simulink library "sensor_processing_libs"  (R2016b)
settings: Solver=VariableStepAuto  StartTime=0.0  StopTime=10.0  RelTol=1e-3
undefined symbols (not defined in the file or in its folder): fsw_params
settings Model: Creator=taylorreynolds  LastModifiedBy=Taylor

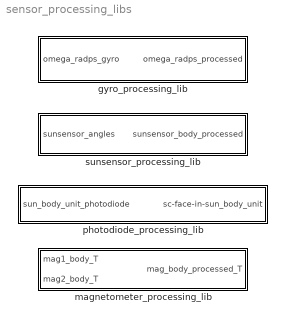
== system sensor_processing_libs ==
  gyro_processing_lib : Subsystem
  magnetometer_processing_lib : Subsystem
  photodiode_processing_lib : Subsystem
  sunsensor_processing_lib : Subsystem

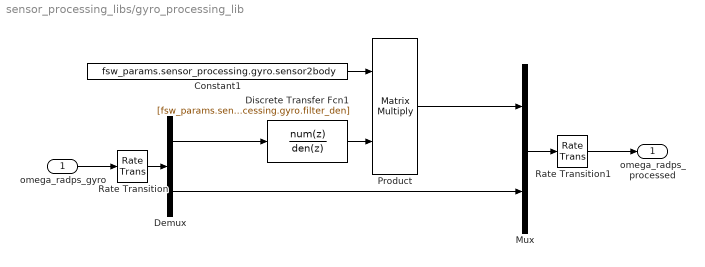
== system sensor_processing_libs/gyro_processing_lib ==
  omega_radps_gyro : Inport
  Constant1 : Constant  Value=fsw_params.sensor_processing.gyro.sensor2body  OutDataTypeStr=single  SampleTime=fsw_params.sensor_processing.gyro.sample_time_s
  Demux : Demux  Outputs=[3 1]
  Discrete Transfer Fcn1 : DiscreteTransferFcn  Numerator=[fsw_params.sensor_processing.gyro.filter_num]  Denominator=[1 fsw_params.sensor_processing.gyro.filter_den]
  Mux : Mux  Inputs=[3 1]
  Product : Product  Multiplication=Matrix(*)
  Rate Transition : RateTransition  OutPortSampleTime=fsw_params.sensor_processing.gyro.sample_time_s
  Rate Transition1 : RateTransition
  omega_radps_processed : Outport
  wires:
  omega_radps_gyro/1 -> Rate Transition/1
  Demux/1 -> Discrete Transfer Fcn1/1
  Constant1/1 -> Product/1
  Demux/2 -> Mux/2
  Discrete Transfer Fcn1/1 -> Product/2
  Rate Transition/1 -> Demux/1
  Rate Transition1/1 -> omega_radps_processed/1
  Mux/1 -> Rate Transition1/1
  Product/1 -> Mux/1

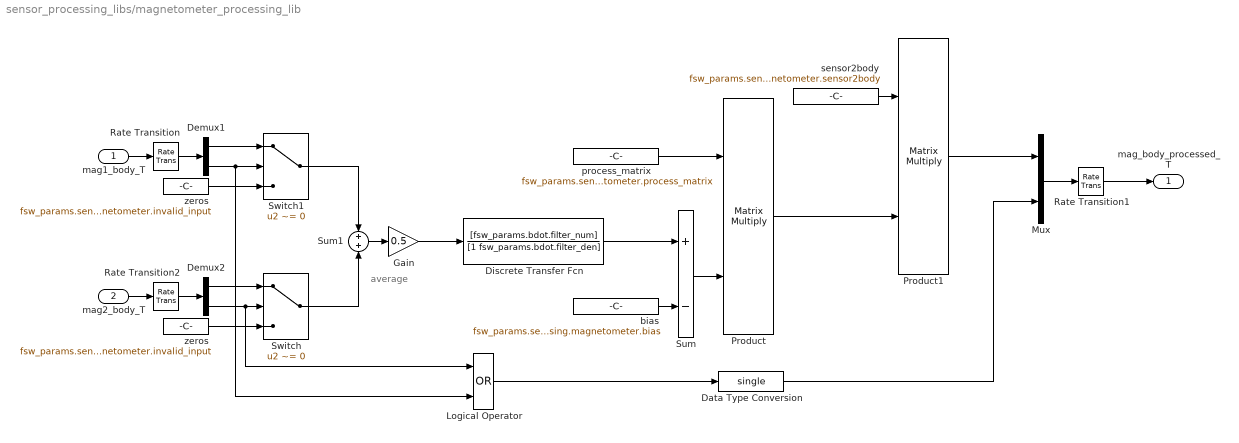
== system sensor_processing_libs/magnetometer_processing_lib ==
  note: average
  mag1_body_T : Inport
  mag2_body_T : Inport  Port=2
  Data Type Conversion : DataTypeConversion  OutDataTypeStr=single
  Demux1 : Demux  Outputs=[3 1]
  Demux2 : Demux  Outputs=[3 1]
  Discrete Transfer Fcn : DiscreteTransferFcn  Numerator=[fsw_params.bdot.filter_num]  Denominator=[1 fsw_params.bdot.filter_den]
  Gain : Gain  Gain=0.5
  Logical Operator : Logic  Operator=OR  AllPortsSameDT=off  OutDataTypeStr=boolean
  Mux : Mux  Inputs=[3 1]
  Product : Product  Multiplication=Matrix(*)
  Product1 : Product  Multiplication=Matrix(*)  OutDataTypeStr=single
  Rate Transition : RateTransition  Deterministic=off  OutPortSampleTime=fsw_params.sensor_processing.magnetometer.sample_time_s
  Rate Transition1 : RateTransition
  Rate Transition2 : RateTransition  Deterministic=off  OutPortSampleTime=fsw_params.sensor_processing.magnetometer.sample_time_s
  Sum : Sum  Inputs=+-
  Sum1 : Sum
  Switch : Switch  Criteria=u2 ~= 0
  Switch1 : Switch  Criteria=u2 ~= 0
  bias : Constant  Value=fsw_params.sensor_processing.magnetometer.bias  OutDataTypeStr=single  SampleTime=fsw_params.sensor_processing.magnetometer.sample_time_s
  process_matrix : Constant  Value=fsw_params.sensor_processing.magnetometer.process_matrix  OutDataTypeStr=single  SampleTime=fsw_params.sensor_processing.magnetometer.sample_time_s
  sensor2body : Constant  Value=fsw_params.sensor_processing.magnetometer.sensor2body  OutDataTypeStr=single  SampleTime=fsw_params.sensor_processing.magnetometer.sample_time_s
  zeros : Constant  Value=fsw_params.sensor_processing.magnetometer.invalid_input  OutDataTypeStr=single  SampleTime=fsw_params.sensor_processing.magnetometer.sample_time_s
  "zeros " : Constant  Value=fsw_params.sensor_processing.magnetometer.invalid_input  OutDataTypeStr=single  SampleTime=fsw_params.sensor_processing.magnetometer.sample_time_s
  mag_body_processed_T : Outport
  wires:
  mag1_body_T/1 -> Rate Transition/1
  bias/1 -> Sum/2
  Sum/1 -> Product/2
  process_matrix/1 -> Product/1
  Discrete Transfer Fcn/1 -> Sum/1
  Product1/1 -> Mux/1
  Product/1 -> Product1/2
  sensor2body/1 -> Product1/1
  Rate Transition1/1 -> mag_body_processed_T/1
  mag2_body_T/1 -> Rate Transition2/1
  Rate Transition/1 -> Demux1/1
  Rate Transition2/1 -> Demux2/1
  Demux1/2 -> Logical Operator/2, Switch1/2
  Demux2/2 -> Logical Operator/1, Switch/2
  Demux2/1 -> Switch/1
  zeros/1 -> Switch/3
  Demux1/1 -> Switch1/1
  "zeros "/1 -> Switch1/3
  Switch/1 -> Sum1/2
  Switch1/1 -> Sum1/1
  Sum1/1 -> Gain/1
  Logical Operator/1 -> Data Type Conversion/1
  Gain/1 -> Discrete Transfer Fcn/1
  Mux/1 -> Rate Transition1/1
  Data Type Conversion/1 -> Mux/2

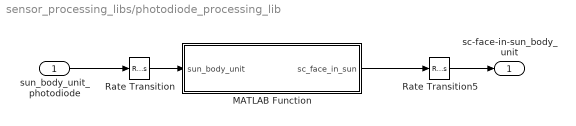
== system sensor_processing_libs/photodiode_processing_lib ==
  sun_body_unit_photodiode : Inport
  MATLAB Function : MATLAB Function  TreatAsAtomicUnit=on
  Rate Transition : RateTransition  OutPortSampleTime=fsw_params.sensor_processing.photodiodes.sample_time_s
  Rate Transition5 : RateTransition
  sc-face-in-sun_body_unit : Outport
  wires:
  sun_body_unit_photodiode/1 -> Rate Transition/1
  MATLAB Function/1(sc_face_in_sun) -> Rate Transition5/1
  Rate Transition/1 -> MATLAB Function/1(sun_body_unit)
  Rate Transition5/1 -> sc-face-in-sun_body_unit/1

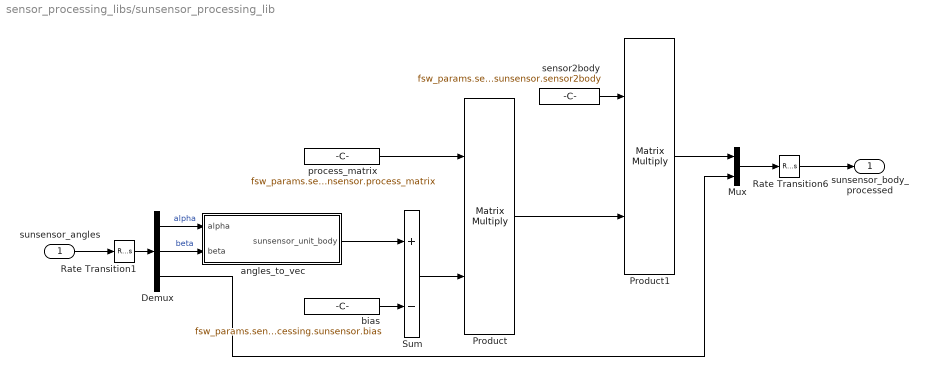
== system sensor_processing_libs/sunsensor_processing_lib ==
  sunsensor_angles : Inport
  Demux : Demux  Outputs=[1 1 1]
  Mux : Mux  Inputs=[3 1]
  Product : Product  Multiplication=Matrix(*)
  Product1 : Product  Multiplication=Matrix(*)
  Rate Transition1 : RateTransition  OutPortSampleTime=fsw_params.sensor_processing.sunsensor.sample_time_s
  Rate Transition6 : RateTransition
  Sum : Sum  Inputs=+-
  angles_to_vec : Subsystem
  bias : Constant  Value=fsw_params.sensor_processing.sunsensor.bias  OutDataTypeStr=single  SampleTime=fsw_params.sensor_processing.sunsensor.sample_time_s
  process_matrix : Constant  Value=fsw_params.sensor_processing.sunsensor.process_matrix  OutDataTypeStr=single  SampleTime=fsw_params.sensor_processing.sunsensor.sample_time_s
  sensor2body : Constant  Value=fsw_params.sensor_processing.sunsensor.sensor2body  OutDataTypeStr=single  SampleTime=fsw_params.sensor_processing.sunsensor.sample_time_s
  sunsensor_body_processed : Outport
  wires:
  process_matrix/1 -> Product/1
  Sum/1 -> Product/2
  Product/1 -> Product1/2
  bias/1 -> Sum/2
  sunsensor_angles/1 -> Rate Transition1/1
  sensor2body/1 -> Product1/1
  Product1/1 -> Mux/1
  Mux/1 -> Rate Transition6/1
  Rate Transition1/1 -> Demux/1
  Rate Transition6/1 -> sunsensor_body_processed/1
  Demux/1 -> angles_to_vec/1(alpha)  "alpha"
  Demux/2 -> angles_to_vec/2(beta)  "beta"
  angles_to_vec/1(sunsensor_unit_body) -> Sum/1
  Demux/3 -> Mux/2

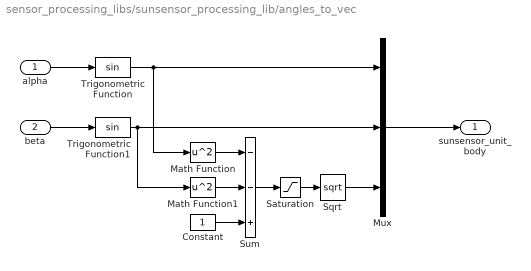
== system sensor_processing_libs/sunsensor_processing_lib/angles_to_vec ==
  alpha : Inport
  beta : Inport  Port=2
  Constant : Constant  OutDataTypeStr=single
  Math Function : Math  Operator=square  SaturateOnIntegerOverflow=on
  Math Function1 : Math  Operator=square  SaturateOnIntegerOverflow=on
  Mux : Mux  Inputs=3
  Saturation : Saturate  UpperLimit=1  LowerLimit=0
  Sqrt : Sqrt  OutputSignalType=real  OutDataTypeStr=single  SaturateOnIntegerOverflow=on
  Sum : Sum  Inputs=--+  OutDataTypeStr=single
  Trigonometric Function : Trigonometry  OutputSignalType=real
  Trigonometric Function1 : Trigonometry  OutputSignalType=real
  sunsensor_unit_body : Outport
  wires:
  alpha/1 -> Trigonometric Function/1
  beta/1 -> Trigonometric Function1/1
  Math Function/1 -> Sum/1
  Trigonometric Function/1 -> Math Function/1, Mux/1
  Math Function1/1 -> Sum/2
  Trigonometric Function1/1 -> Math Function1/1, Mux/2
  Constant/1 -> Sum/3
  Sum/1 -> Saturation/1
  Sqrt/1 -> Mux/3
  Mux/1 -> sunsensor_unit_body/1
  Saturation/1 -> Sqrt/1

== matlab function sensor_processing_libs/photodiode_processing_lib/MATLAB Function ==
  data: sun_body_unit input; sc_face_in_sun output
 function sc_face_in_sun = fcn(sun_body_unit)

body_vecs   = [ 1  0  0;
                0  1  0;
                0  0  1;
               -1  0  0;
                0 -1  0 ];
            
num_faces = 5;
dot_prods   = zeros(1,5);

for i = 1:num_faces
    dot_prods(i)    = dot(sun_body_unit,body_vecs(i,:));
end

[val,axis] = max(dot_prods);

if val < 0
    % this is only the case if the PPT is pointing right at the sun
    sc_face_in_sun = [ 0 0 -1 ]';
else
    sc_face_in_sun  = body_vecs(axis,:)';
end
